simulink model "model_math_Hoang_Phuc"  (R2019a)
settings: Solver=FixedStepAuto  StartTime=0.0  StopTime=10.0  FixedStep=0.01  RelTol=1e-3
undefined symbols (not defined in the file): K
settings Model: Creator=chute  LastModifiedBy=chute

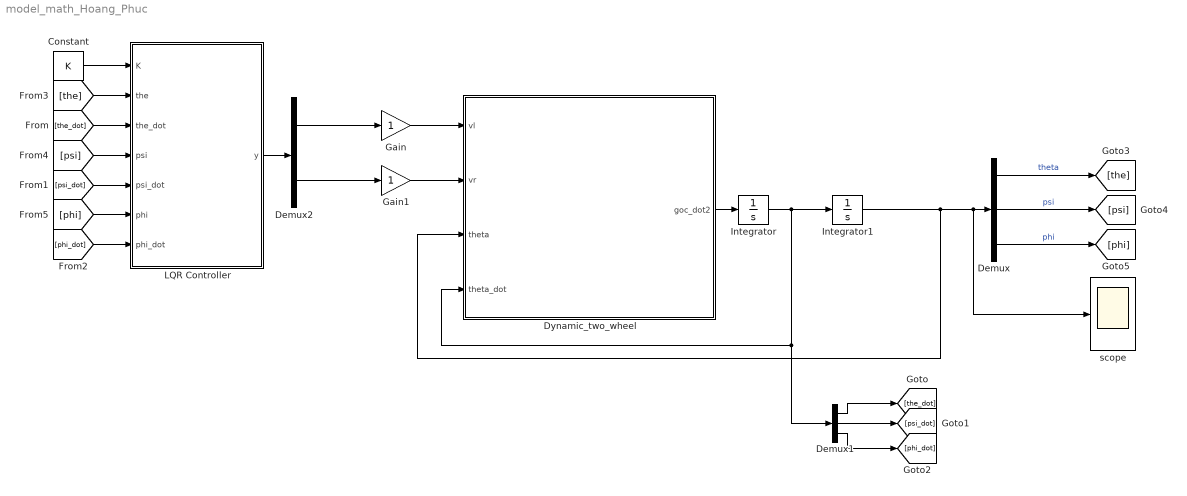
== system model_math_Hoang_Phuc ==
  Constant : Constant  Value=K
  Demux : Demux  Outputs=3
  Demux1 : Demux  Outputs=3
  Demux2 : Demux  Outputs=2
  Dynamic_two_wheel : MATLAB Function  TreatAsAtomicUnit=on
  Gain : Gain
  Gain1 : Gain
  Integrator : Integrator  InitialCondition=[0.01;0.01;0.01]
  Integrator1 : Integrator  InitialCondition=[0.01;0.01;0.01]
  "LQR Controller " : MATLAB Function  TreatAsAtomicUnit=on
  scope : Scope
  wires:
  Demux2/2 -> Gain1/1
  Gain1/1 -> Dynamic_two_wheel/2(vr)
  [phi] -> "LQR Controller "/6(phi)
  Gain/1 -> Dynamic_two_wheel/1(vl)
  Constant/1 -> "LQR Controller "/1(K)
  "LQR Controller "/1(y) -> Demux2/1
  [the] -> "LQR Controller "/2(the)
  Integrator/1 -> Integrator1/1, Dynamic_two_wheel/4(theta_dot), Demux1/1
  [psi] -> "LQR Controller "/4(psi)
  [psi_dot] -> "LQR Controller "/5(psi_dot)
  Demux1/2 -> [psi_dot]
  [the_dot] -> "LQR Controller "/3(the_dot)
  Demux2/1 -> Gain/1
  Dynamic_two_wheel/1(goc_dot2) -> Integrator/1
  Demux1/3 -> [phi_dot]
  [phi_dot] -> "LQR Controller "/7(phi_dot)
  Demux/3 -> [phi]  "phi"
  Integrator1/1 -> Dynamic_two_wheel/3(theta), scope/1, Demux/1
  Demux/1 -> [the]  "theta"
  Demux/2 -> [psi]  "psi"
  Demux1/1 -> [the_dot]

== matlab function model_math_Hoang_Phuc/Dynamic_two_wheel ==
  data: vl input; vr input; goc_dot2 output; theta input; theta_dot input
function goc_dot2 = fcn(vl,vr,theta,theta_dot)
%% declare the parameter
g =9.81; % gravity acceleration
m =0.044; % wheel weight
R =0.0267; % Wheel radius
M =0.92;  % body weight
W =0.145; % Body width
D =0.055; % Body depth
H =0.185;% Body Height
L =0.1;% distance
J_psi  = M*L^2/3; % Body inertia moment
Jw = m*R^2/2;  %Wheel inertia moment
J_phi = M*(W^2+D^2)/12; % Body yaw inertia moment
Jm =1.47*10^(-5); % Dc motor inertia moment
Rm = 40; % Dc motor resitance
Kb = 0.0218; % DC motor EMF
Kt = 0.0197; % DC motor torque const
fm = 0.0022; % friction cof between body and DC motor.
fw = 0; % friction cof between wheel and floor



n =30 ; %gear ratio
anp = n*Kt/Rm;
bet = n*Kt*Kb/Rm +fm;

the = theta(1);
psi = theta(2);
phi = theta(3);

the_dot = theta_dot(1);
psi_dot = theta_dot(2);
phi_dot = theta_dot(3);


F_the = anp*(vl+vr)-2*(bet+fw)*the_dot+2*bet*psi_dot;
F_psi = -anp*(vl+vr)+2*bet*the_dot-2*bet*psi_dot;
F_phi = W*anp*(vr-vl)/(2*R)-W^2*((bet+fw)*phi_dot)/2*R^2;
tor =[F_the;F_psi;F_phi];

M1 = ...
[2*Jw + 2*Jm*n^2 + R^2*(M + 2*m),  L*M*R*cos(psi)-2*Jm*n^2,          0;
       L*M*R*cos(psi) - 2*Jm*n^2, J_psi + L^2*M + 2*Jm*n^2,          0;
 0,0,J_phi + (W^2*m)/2 + L^2*M*sin(psi)^2 + (W^2*(Jw + Jm*n^2))/(2*R^2)];


C = ...
[0,-L*M*R*psi_dot*sin(psi),0;
 0,0,-L^2*M*phi_dot*cos(psi)*sin(psi);
 0,L^2*M*phi_dot*cos(psi)*sin(psi),L^2*M*psi_dot*cos(psi)*sin(psi)];


G=...
[0;
 -L*M*g*sin(psi);
 0];
dei = transpose([the_dot  psi_dot  phi_dot]);

goc_dot2 = inv(M1)*(tor-C*dei-G);

== matlab function model_math_Hoang_Phuc/LQR Controller  ==
  data: K input; y output; the input; the_dot input; psi input; psi_dot input; phi input; phi_dot input
function y = fcn(K,the, the_dot, psi,psi_dot, phi, phi_dot)
XXX = [the;the_dot; psi;psi_dot; phi; phi_dot];
y = -K*XXX;
